simulink model "sldemo_mdlref_house"  (Simulink 7.6)
settings: Solver=ode3  SolverMode=SingleTasking  StartTime=0.0  StopTime=2*24*60*60  FixedStep=60  RelTol=1e-3  AbsTol=1e-6
model workspace (MAT data in the model file):
  Req = 0.00153711229591
  c = 1005.4
  M = 1778.36911446
  TinIC = 20
PreLoadFcn:
  | thermdat
settings Model: Creator=The MathWorks Inc.  ExtModeAutoUpdateStatusClock=off
settings DataIOCC: ExternalInput=[]  InitialState=[]  LimitDataPoints=off  SaveOutput=off  SaveTime=off
settings OptimizationCC: BlockReduction=off  BooleanDataType=off  InlineParams=on  InlineInvariantSignals=on  InitFltsAndDblsToZero=on
settings DebuggingCC: SaveWithParameterizedLinksMsg=none  CheckExecutionContextPreStartOutputMsg=on  CheckExecutionContextRuntimeOutputMsg=on  SolverPrmCheckMsg=none  MultiTaskDSMMsg=warning  MultiTaskCondExecSysMsg=none  SigSpecEnsureSampleTimeMsg=none  IntegerOverflowMsg=none
settings HardwareCC: TargetHWDeviceType=32-bit Generic
settings ModelReferenceCC: ModelReferenceMinAlgLoopOccurrences=on
settings RTWCC: IncludeERTFirstTime=on
settings CodeAppCC: MaxIdLength=100
settings GRTTargetCC: TargetFcnLib=ansi_tfl_tmw.mat

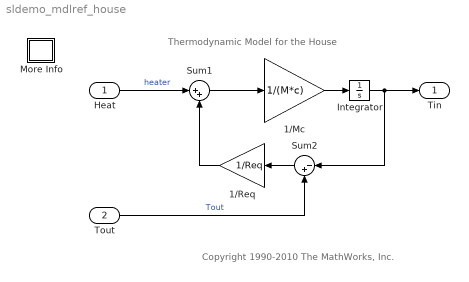
== system sldemo_mdlref_house ==
  note: Thermodynamic Model
      | for the House
  note: Copyright 1990-2010 The MathWorks, Inc.
  Heat : Inport  OutDataTypeStr=double  PortDimensions=1  SampleTime=0
  Tout : Inport  Port=2  OutDataTypeStr=double  PortDimensions=1  SampleTime=0
  1/Mc : Gain  Gain=1/(M*c)  SaturateOnIntegerOverflow=on  OutDataTypeStr=Inherit: Same as input  ParamDataTypeStr=Inherit: Same as input
  1/Req : Gain  Gain=1/Req  SaturateOnIntegerOverflow=on  OutDataTypeStr=Inherit: Same as input  ParamDataTypeStr=Inherit: Same as input
  Integrator : Integrator  InitialCondition=TinIC
  More Info : Subsystem
      settings: OpenFcn=showdemo('sldemo_mdlref_depgraph')
      mask Display: disp('?')
  Sum1 : Sum  Inputs=|++  SaturateOnIntegerOverflow=on  InputSameDT=on  OutDataTypeStr=Inherit: Same as first input
  Sum2 : Sum  Inputs=|-+  SaturateOnIntegerOverflow=on  InputSameDT=on  OutDataTypeStr=Inherit: Same as first input
  Tin : Outport  InitialOutput=0
  wires:
  Integrator/1 -> Tin/1, Sum2/1
  1/Mc/1 -> Integrator/1
  1/Req/1 -> Sum1/2
  Sum2/1 -> 1/Req/1
  Sum1/1 -> 1/Mc/1
  Heat/1 -> Sum1/1  "heater"
  Tout/1 -> Sum2/2  "Tout"

== system sldemo_mdlref_house/More Info ==
